simulink model "MSFartoystyring2017"  (R2017a)
settings: Solver=ode45  StartTime=tstart  StopTime=tstop  RelTol=1e-3  EnableMultiTasking=on
undefined symbols (not defined in the file): c, k_d_dc, k_i_nc, k_p_dc, k_p_nc, msfartoystyring, p0, psi0, r0, tsamp, v0
libraries: dsparch4 x1, simulink x1
settings Model: ExtModeAutoUpdateStatusClock=off  Creator=christh  LastModifiedBy=Martin
settings DataIOCC: LimitDataPoints=on  SaveFormat=Array  SignalLoggingSaveFormat=ModelDataLogs
settings OptimizationCC: ExpressionDepthLimit=2147483647  InitFltsAndDblsToZero=on  LifeSpan=inf
settings DebuggingCC: UnderspecifiedInitializationDetection=Classic  MergeDetectMultiDrivingBlocksExec=none  SolverPrmCheckMsg=warning  FcnCallInpInsideContextMsg=warning  StateNameClashWarn=warning  SFUnexpectedBacktrackingDiag=warning  SFNoUnconditionalDefaultTransitionDiag=warning  SFExecutionAtInitializationDiag=none
settings HardwareCC: ProdBitPerPointer=32  ProdBitPerSizeT=32  ProdBitPerPtrDiffT=32  ProdLargestAtomicFloat=None  ProdIntDivRoundTo=Undefined  ProdEndianess=Unspecified  ProdWordSize=32  ProdHWDeviceType=32-bit Generic
settings ModelReferenceCC: PropagateSignalLabelsOutOfModel=off
settings GRTTargetCC: TargetLangStandard=C89/C90 (ANSI)  GeneratePreprocessorConditionals=Disable all  CombineOutputUpdateFcns=off  GRTInterface=on
settings ConfigComp: CovMetricSettings=dw  CovHtmlReporting=on  CovSaveCumulativeToWorkspaceVar=on  CovSaveSingleToWorkspaceVar=on  CovExternalEMLEnable=off

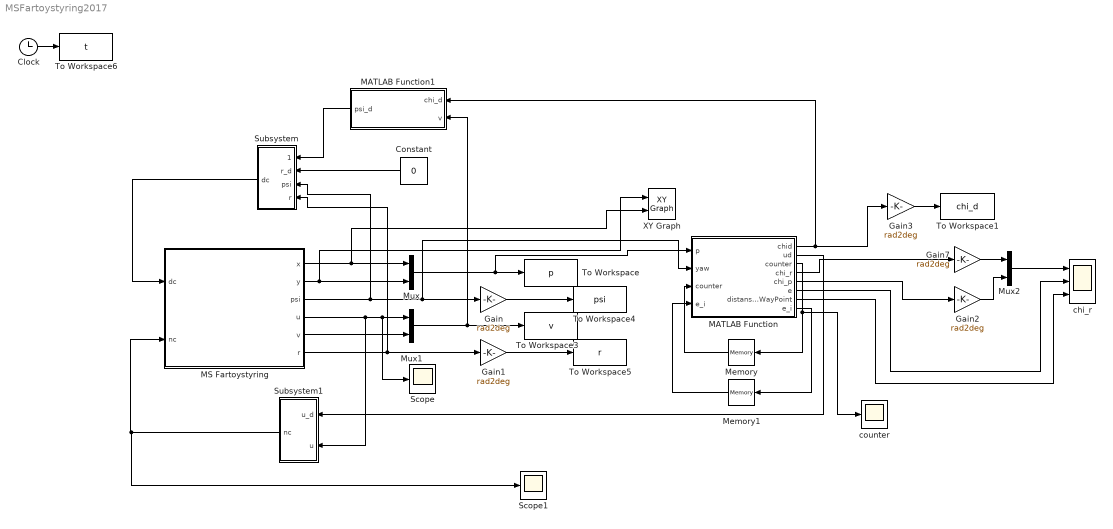
== system MSFartoystyring2017 ==
  Clock : Clock
  Constant : Constant  Value=0
  Gain{,1..3,7} (5 alike) : Gain  Gain=rad2deg
  MATLAB Function : MATLAB Function  TreatAsAtomicUnit=on
  MATLAB Function1 : MATLAB Function  TreatAsAtomicUnit=on
  MS Fartoystyring : Subsystem  mask(MS Fartoystyring for Assignment 3 G&C){x0=p0(1), y0=p0(2), u0=v0(1), v0=v0(2), psi0=psi0, r0=r0, c=c}
      mask prompts: x0 "x(t0) (m)"; y0 "y(t0) (m)"; u0 "u(t0) (m/s)"; v0 "v(t0) (m/s)"; psi0 "psi(t0) (rad)"; r0 "r(t0) (rad/s)"; c "current (0 or 1)"
      mask help:
      | Block corresponding to Figure 1 in the assignment text. Gives the response of the ship.
      |
      | The design speed of MS Fartoystyring is u=8.23 m/s.
      |
      | Input:
      | dc: commanded rudder (rad), dmax=25*pi/180
      | nc: commanded shaft speed (rad/s), nmax=85*2*pi/60
      |
      | Output:
      | x: north pos (m)
      | y: east pos (m)
      | u: surge (m/s)
      | v: sway (m/s)
      | psi: heading (rad)
      | r: yaw (rad/s)
      mask Help: Comments, bugs and help requests can be directed to the TA. Email on course website.
  Memory : Memory  X0=1
  Memory1 : Memory
  Mux : Mux  Inputs=2
  Mux1 : Mux  Inputs=2
  Mux2 : Mux  Inputs=2
  Scope : Scope
  Scope1 : Scope
  Subsystem : Subsystem
  Subsystem1 : Subsystem
  To Workspace : ToWorkspace  VariableName=p  SampleTime=tsamp
  To Workspace1 : ToWorkspace  VariableName=chi_d  SampleTime=tsamp
  To Workspace3 : ToWorkspace  VariableName=v  SampleTime=tsamp
  To Workspace4 : ToWorkspace  VariableName=psi  SampleTime=tsamp
  To Workspace5 : ToWorkspace  VariableName=r  SampleTime=tsamp
  To Workspace6 : ToWorkspace  VariableName=t  SampleTime=tsamp
  XY Graph : simulink/Sinks/XY Graph  xmin=-10000  xmax=10000  ymin=-10000  ymax=10000  st=-1
  chi_r : Scope  NumInputPorts=3
  counter : Scope
  wires:
  Clock/1 -> To Workspace6/1
  MS Fartoystyring/1(x) -> XY Graph/2, Mux/1
  MS Fartoystyring/2(y) -> XY Graph/1, Mux/2
  MS Fartoystyring/4(u) -> Subsystem1/2(u), Scope/1, Mux1/1
  MS Fartoystyring/5(v) -> Mux1/2
  Mux/1 -> MATLAB Function/1(p), To Workspace/1
  Mux1/1 -> MATLAB Function1/2(v), To Workspace3/1
  MS Fartoystyring/3(psi) -> Subsystem/3(psi), MATLAB Function/2(yaw), Gain/1
  Subsystem1/1(nc) -> Scope1/1, MS Fartoystyring/2(nc)
  Gain/1 -> To Workspace4/1
  Subsystem/1(dc) -> MS Fartoystyring/1(dc)
  MS Fartoystyring/6(r) -> Subsystem/4(r), Gain1/1
  Gain1/1 -> To Workspace5/1
  MATLAB Function/2(ud) -> Subsystem1/1(u_d)
  MATLAB Function/3(counter) -> Memory/1, counter/1
  Memory/1 -> MATLAB Function/3("counter ")
  Constant/1 -> Subsystem/2(r_d)
  Gain7/1 -> Mux2/1
  MATLAB Function/4(chi_r) -> Gain7/1
  MATLAB Function/6(e) -> chi_r/2
  MATLAB Function/5(chi_p) -> Gain2/1
  Gain2/1 -> Mux2/2
  Mux2/1 -> chi_r/1
  MATLAB Function/7(distansToWayPoint) -> chi_r/3
  MATLAB Function/8(e_i) -> Memory1/1
  Memory1/1 -> MATLAB Function/4("e_i ")
  MATLAB Function/1(chid) -> Gain3/1, MATLAB Function1/1(chi_d)
  Gain3/1 -> To Workspace1/1
  MATLAB Function1/1(psi_d) -> Subsystem/1(psi_d)

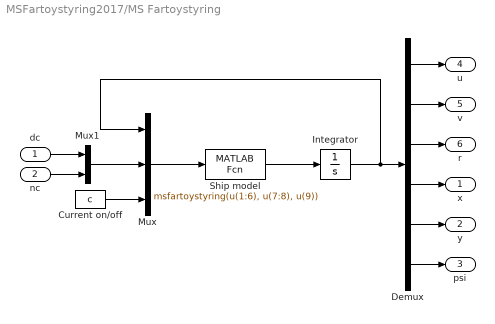
== system MSFartoystyring2017/MS Fartoystyring ==
  dc : Inport
  nc : Inport  Port=2
  Current on/off : Constant  Value=c
  Demux : Demux  Outputs=6
  Integrator : Integrator  InitialCondition=[u0 v0 r0 x0 y0 psi0]'
  Mux : Mux  Inputs=3
  Mux1 : Mux  Inputs=2
  Ship model : MATLABFcn  MATLABFcn=msfartoystyring(u(1:6), u(7:8), u(9))  OutputDimensions=6
  x : Outport
  y : Outport  Port=2
  psi : Outport  Port=3
  u : Outport  Port=4
  v : Outport  Port=5
  r : Outport  Port=6
  wires:
  Integrator/1 -> Mux/1, Demux/1
  Mux1/1 -> Mux/2
  dc/1 -> Mux1/1
  nc/1 -> Mux1/2
  Demux/1 -> u/1
  Demux/2 -> v/1
  Demux/3 -> r/1
  Demux/4 -> x/1
  Demux/5 -> y/1
  Demux/6 -> psi/1
  Current on/off/1 -> Mux/3
  Ship model/1 -> Integrator/1
  Mux/1 -> Ship model/1

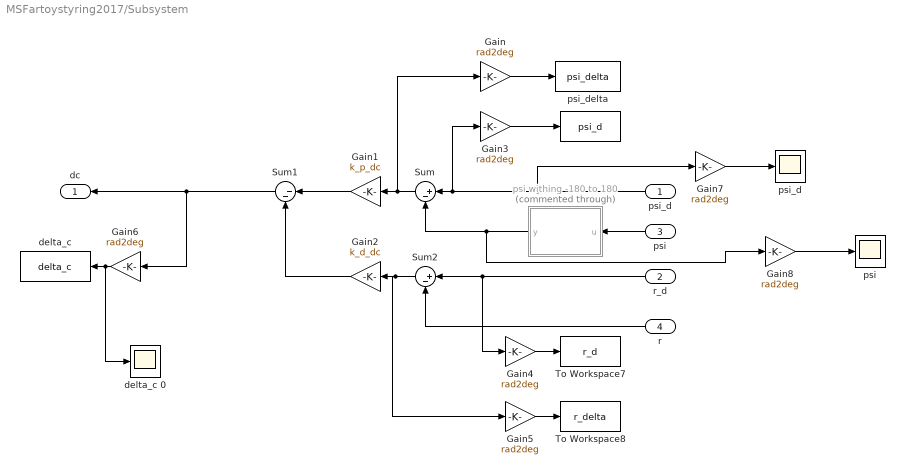
== system MSFartoystyring2017/Subsystem ==
  psi_d : Inport
  r_d : Inport  Port=2
  psi : Inport  Port=3
  r : Inport  Port=4
  " " : ToWorkspace  VariableName=psi_d  SampleTime=tsamp
  Gain{,3..8} (7 alike) : Gain  Gain=rad2deg
  Gain1 : Gain  Gain=k_p_dc
  Gain2 : Gain  Gain=k_d_dc
  Sum : Sum  Inputs=|+-
  Sum1 : Sum  Inputs=|--
  Sum2 : Sum  Inputs=|+-
  To Workspace7 : ToWorkspace  VariableName=r_d  SampleTime=tsamp
  To Workspace8 : ToWorkspace  VariableName=r_delta  SampleTime=tsamp
  delta_c : ToWorkspace  VariableName=delta_c  SampleTime=tsamp
  delta_c 0 : Scope
  "psi " : Scope
  psi withing -180 to 180 : MATLAB Function  Commented=through  TreatAsAtomicUnit=on
  "psi_d " : Scope
  psi_delta : ToWorkspace  VariableName=psi_delta  SampleTime=tsamp
  dc : Outport
  wires:
  r_d/1 -> Gain4/1, Sum2/1
  psi_d/1 -> Gain7/1, Gain3/1, Sum/1
  Sum/1 -> Gain/1, Gain1/1
  Gain2/1 -> Sum1/2
  Gain1/1 -> Sum1/1
  Sum2/1 -> Gain5/1, Gain2/1
  psi/1 -> psi withing -180 to 180/1(u)
  r/1 -> Sum2/2
  Gain/1 -> psi_delta/1
  Gain3/1 -> " "/1
  Gain4/1 -> To Workspace7/1
  Gain5/1 -> To Workspace8/1
  Sum1/1 -> Gain6/1, dc/1
  Gain6/1 -> delta_c 0/1, delta_c/1
  psi withing -180 to 180/1(y) -> Gain8/1, Sum/2
  Gain7/1 -> "psi_d "/1
  Gain8/1 -> "psi "/1

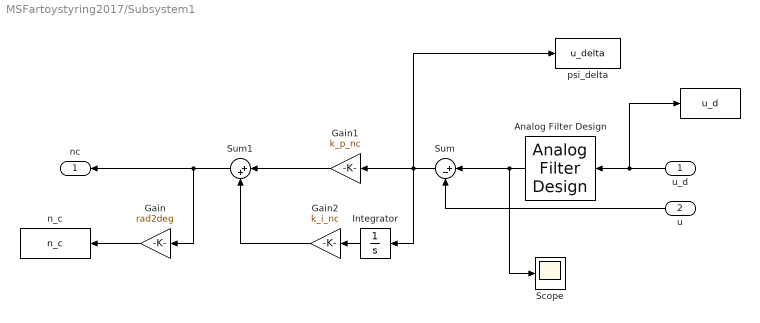
== system MSFartoystyring2017/Subsystem1 ==
  u_d : Inport
  u : Inport  Port=2
  " " : ToWorkspace  VariableName=u_d  SampleTime=tsamp
  Analog Filter Design : dsparch4/Analog Filter Design  method=Butterworth  filttype=Lowpass  N=1  Wlo=1/150  Whi=80  Rp=2  Rs=40
  Gain : Gain  Gain=rad2deg
  Gain1 : Gain  Gain=k_p_nc
  Gain2 : Gain  Gain=k_i_nc
  Integrator : Integrator  LimitOutput=on  UpperSaturationLimit=85*2*pi/60  LowerSaturationLimit=-85*2*pi/60
  Scope : Scope
  Sum : Sum  Inputs=|+-
  Sum1 : Sum  Inputs=|++
  n_c : ToWorkspace  VariableName=n_c  SampleTime=tsamp
  psi_delta : ToWorkspace  VariableName=u_delta  SampleTime=tsamp
  nc : Outport
  wires:
  u/1 -> Sum/2
  Sum/1 -> Integrator/1, Gain1/1, psi_delta/1
  u_d/1 -> " "/1, Analog Filter Design/1
  Sum1/1 -> Gain/1, nc/1
  Gain1/1 -> Sum1/1
  Gain2/1 -> Sum1/2
  Integrator/1 -> Gain2/1
  Analog Filter Design/1 -> Scope/1, Sum/1
  Gain/1 -> n_c/1

== matlab function MSFartoystyring2017/Subsystem/psi withing -180 to 180 ==
  data: u input; y output
function y = boundedPsi(u)

u = mod(u,pi*2);
if u > pi
    u = u-2*pi;
end
y = u;

== matlab function MSFartoystyring2017/MATLAB Function ==
  data: p input; yaw input; chid output; counter input; ud output; counter output; chi_r output; chi_p output; e output; distansToWayPoint output; e_i input; e_i output
function [chid,ud,counter,chi_r,chi_p,e,distansToWayPoint,e_i] = fcn(p,yaw,counter,e_i)

wp = [0 -3500 -7000 -12000 -15000 -18000;0 -2500 -500 -3500 -500 -2000];

distansToWayPoint = sqrt((p(1)-wp(1,counter+1))^2+(p(2)-wp(2,counter+1))^2);
if distansToWayPoint < 100
    counter = counter +1;
end
k_p = 0.00083; %må vær mindre en 0.0009
k_i = 0.0000025;
%R = 5000;
%delta = 100;
%chi_p = acos((wp(1,counter)-wp(1,counter+1))/sqrt((wp(1,counter+1)-wp(1,counter))^2+(wp(2,counter+1)-wp(2,counter))^2));
chi_p = atan2(wp(2,counter+1)-wp(2,counter),wp(1,counter+1)-wp(1,counter));
% if (wp(2,counter) > wp(2,counter+1)) && (wp(1,counter) > wp(1,counter+1))
%     chi_p = chi_p-pi;
% elseif (wp(1,counter+1) < wp(1,counter)) && (wp(2,counter+1) > wp(2,counter))
%     chi_p = chi_p-pi;
% end
% if wp(2,counter) > wp(2,counter+1)
%     chi_p = chi_p-pi;
% end
h = 0.01;
e = -(p(1)-wp(1,counter))*sin(chi_p)+(p(2)-wp(2,counter))*cos(chi_p);
e_i = e_i + e*h;

chi_r = atan(-e*k_p-e_i*k_i);

% if chi_p < 0
%     chid 

chid = chi_p-chi_r;
% else 
%     chid = chi_p + chi_r;
% end
chid = chi_p + chi_r;

% chi_r = 0;
% chid = acos(e/(sqrt(e^2+delta^2))) - pi/2+chi_p;
% 
chid = mod(chid,pi*2);
if chid > pi
    chid = -2*pi + chid;
end

if yaw > pi/2 && chid < -pi/2
    chid = chid+2*pi;
elseif yaw < -pi/2 && chid > pi/2
    chid = chid-2*pi;
end 
    
ud = 6.63;

== matlab function MSFartoystyring2017/MATLAB Function1 ==
  data: chi_d input; psi_d output; v input
function psi_d = courseToYaw(chi_d,v)
U = sqrt(v(1)^2+v(2)^2);
beta = asin(v(2)/U);


psi_d = chi_d - beta;
